simulink model "MPC_design_2out"  (R2019b)
settings: Solver=FixedStepAuto  StartTime=0.0  StopTime=Time(end)  FixedStep=Time(2)  RelTol=1e-3
values from neighbouring files (symbols this model uses):
  Aa = [aa11 aa12 aa13 aa14 ... (first row only)    [model_generate.m]    (also in mpc_2states_working.mat = [-1.60846560847 15.8608695652 167280.42328 290539.68254 -1.1)
  Bb = [bb11 bb12 ... (first row only)    [model_generate.m]    (also in mpc_2states_working.mat = [1.60846560847  0; 15.8608695652  0; -61121.6931217  38000; )
  Cc = [1 0 0 0; 0 1 0 0]    [model_generate.m]    (also in mpc_2states_working.mat = [1  0  0  0; 0  1  0  0])
  Dd = zeros(2)    [model_generate.m]    (also in mpc_2states_working.mat = [0  0; 0  0])
libraries: mpclib x1
settings Model: Creator=shouv  LastModifiedBy=shouv

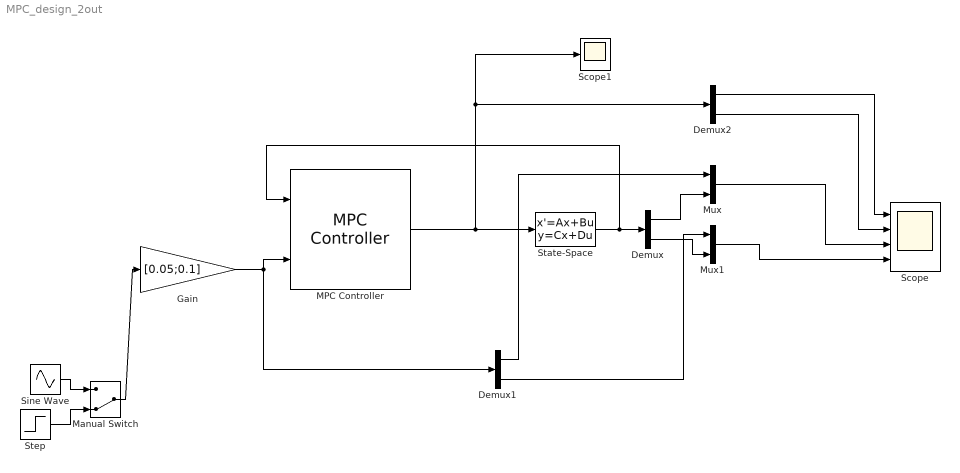
== system MPC_design_2out ==
  Demux : Demux  Outputs=2
  Demux1 : Demux  Outputs=2
  Demux2 : Demux  Outputs=2
  Gain : Gain  Gain=[0.05;0.1]
  MPC Controller : mpclib/MPC Controller  SCDEnableBlockLinearizationSpecification=on  mpcobj=mpc1  is_multiple=0  enable_value=0  return_u0=off  updateMPCinCallerWorkspace=on  md_inport=off  mv_inport=off  uref_inport=off  return_cost=off  return_mvseq=off  return_qpstatus=off  return_xseq=off  return_state=off  return_ovseq=off  state_inport=off  umin_inport=off  umax_inport=off  ymin_inport=off  ymax_inport=off  cc_inport=off  ywt_inport=off  uwt_inport=off  duwt_inport=off  rhoeps_inport=off  pm_inport=off  MaximumP=10  HorizonChoice=FixedHorizon  n_ts=0.025  n_p=14  n_mv=2  n_md=0  n_ud=0  n_mo=2  n_uo=0  BlockDataType=double  SampleTimeInherited=off  switch_inport=off
  Manual Switch : ManualSwitch  CurrentSetting=0
  Mux : Mux  Inputs=2
  Mux1 : Mux  Inputs=2
  Scope : Scope  NumInputPorts=4
  Scope1 : Scope
  Sine Wave : Sin  SampleTime=0
  State-Space : StateSpace  A=Aa  B=Bb  C=Cc  D=Dd  InitialCondition=0
  Step : Step  SampleTime=0
  wires:
  MPC Controller/1 -> Demux2/1, Scope1/1, State-Space/1
  State-Space/1 -> Demux/1, MPC Controller/1
  Gain/1 -> Demux1/1, MPC Controller/2
  Demux/1 -> Mux/2
  Demux/2 -> Mux1/2
  Demux1/1 -> Mux/1
  Demux1/2 -> Mux1/1
  Mux/1 -> Scope/3
  Mux1/1 -> Scope/4
  Demux2/2 -> Scope/2
  Demux2/1 -> Scope/1
  Sine Wave/1 -> Manual Switch/1
  Step/1 -> Manual Switch/2
  Manual Switch/1 -> Gain/1
